simulink model "BAM"  (R2025b)
settings: Solver=FixedStepAuto  StartTime=0.0  StopTime=SimPar.model_params.stop_time  RelTol=1e-3
libraries: simulink x1
settings Model: Creator=macheson  LastModifiedBy=wyatt

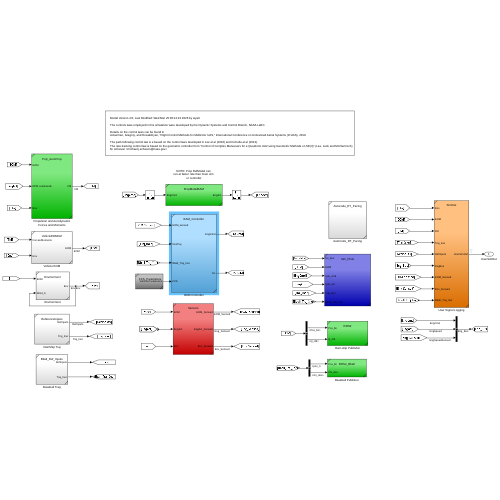
[thumbnail: Simulink's stored preview of the top-level diagram]
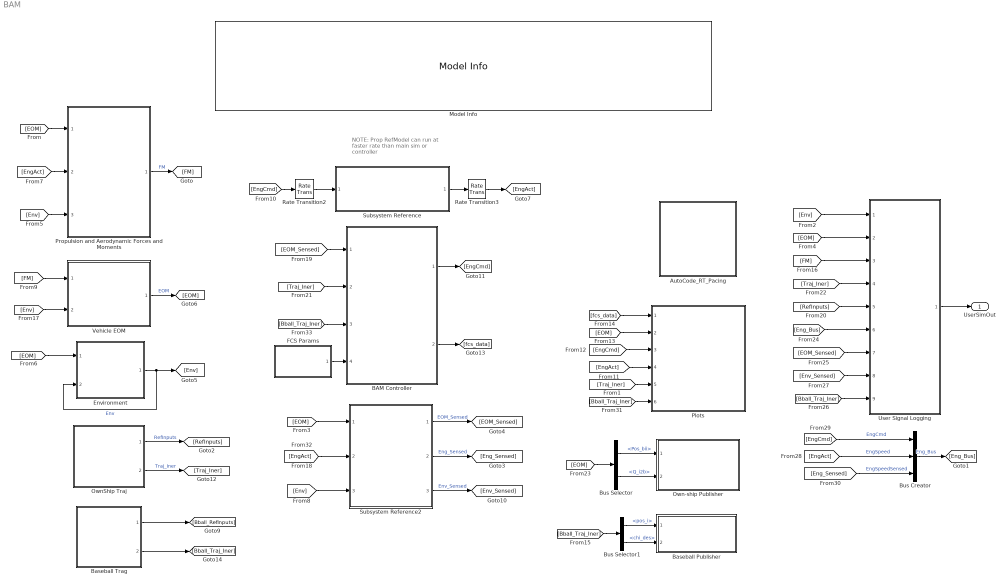
== system BAM ==
  note: NOTE: Prop RefModel can
      | run at faster rate than main sim
      | or controller
  AutoCode_RT_Pacing : Subsystem  ReferencedSubsystem=Autocode_RT_Pacing
  BAM Controller : Subsystem  ReferencedSubsystem=BAM_Controller
  Baseball Publisher : Subsystem  ReferencedSubsystem=ROS2_Bball
  Baseball Trag : Subsystem  ReferencedSubsystem=Bball_Ref_Inputs
  Bus Creator : BusCreator  Inputs=3  OutDataTypeStr=Bus: BUS_PROP_CMD
  Bus Selector : BusSelector  OutputSignals=InertialData.Pos_bii,InertialData.Q_i2b
  Bus Selector1 : BusSelector  OutputSignals=pos_i,chi_des
  Environment : Subsystem  ReferencedSubsystem=Environment
  FCS Params : Subsystem  ReferencedSubsystem=FCS_Parameters
  Model Info : simulink/Model-Wide Utilities/Model Info  Frame=on  DisplayStringWithTags=|  HorizontalTextAlignment=Left  LeftAlignmentValue=0.02
      | Model Version %<ModelVersion>; Last Modified: %<LastModificationDate> by %<LastModifiedBy>
      | 
      | The controls laws employed in this simulation were developed by the Dynamic Systems and Control Branch, NASA LaRC.
      | 
      | Details on the control laws can be found in
      | Ackerman, Gregory, and Hovakimyan, "Flight Control Methods for Multirotor UAS," International Conference on Unmanned Aerial Systems (ICUAS), 2019.
      | 
      | The path-following control law is a based on the control laws developed in Lee et al (2010) and Cichella et al (2013). 
      | The rate-tracking control law is based on the geometric controller from "Control of Complex Maneuvers for a Quadrotor UAV using Geometric Methods on SE(3)" (Lee, Leok and McClamroch)
      | M. Acheson <michael.j.acheson@nasa.gov>
  Own-ship Publisher : Subsystem  ReferencedSubsystem=ROS2
  OwnShip Traj : Subsystem  ReferencedSubsystem=ReferenceInputs
  Plots : Subsystem  ReferencedSubsystem=Sim_Plots
  Propulsion and Aerodynamic Forces and Moments : Subsystem  ReferencedSubsystem=Poly_AeroProp
  Rate Transition2 : RateTransition  OutPortSampleTime=SimIn.model_params.sim_rate
  Rate Transition3 : RateTransition  OutPortSampleTime=SimIn.model_params.sim_rate
  Subsystem Reference : Subsystem  ReferencedSubsystem=PropModelBAM
  Subsystem Reference2 : Subsystem  ReferencedSubsystem=Sensors
  User Signal Logging : Subsystem  ReferencedSubsystem=SimOut
  Vehicle EOM : Subsystem  ReferencedSubsystem=VehicleEOMRef
  UserSimOut : Outport
  wires:
  Vehicle EOM/1 -> [EOM]  "EOM"
  [FM] -> Vehicle EOM/1
  [Env] -> Vehicle EOM/2
  [EOM] -> Propulsion and Aerodynamic Forces and Moments/1
  OwnShip Traj/1 -> [RefInputs]  "RefInputs"
  Propulsion and Aerodynamic Forces and Moments/1 -> [FM]  "FM"
  [EOM] -> Subsystem Reference2/1
  Environment/1 -> Environment/2, [Env]  "Env"
  [EOM] -> Environment/1
  Subsystem Reference/1 -> Rate Transition3/1
  [EngCmd] -> Rate Transition2/1
  [EngAct] -> Plots/4
  [EngCmd] -> Plots/3
  [EOM] -> Plots/2
  [fcs_data] -> Plots/1
  [EngAct] -> Propulsion and Aerodynamic Forces and Moments/2
  Rate Transition2/1 -> Subsystem Reference/1
  Rate Transition3/1 -> [EngAct]
  Subsystem Reference2/2 -> [Eng_Sensed]  "Eng_Sensed"
  Subsystem Reference2/3 -> [Env_Sensed]  "Env_Sensed"
  [Env] -> Subsystem Reference2/3
  [EngAct] -> Subsystem Reference2/2
  Subsystem Reference2/1 -> [EOM_Sensed]  "EOM_Sensed"
  FCS Params/1 -> BAM Controller/4
  [EOM_Sensed] -> BAM Controller/1
  [Traj_Iner] -> BAM Controller/2
  BAM Controller/1 -> [EngCmd]
  OwnShip Traj/2 -> [Traj_Iner]  "Traj_Iner"
  BAM Controller/2 -> [fcs_data]
  [Env] -> User Signal Logging/1
  [EOM] -> User Signal Logging/2
  [Env_Sensed] -> User Signal Logging/8
  [EOM_Sensed] -> User Signal Logging/7
  [Eng_Bus] -> User Signal Logging/6
  [Traj_Iner] -> User Signal Logging/4
  [RefInputs] -> User Signal Logging/5
  [FM] -> User Signal Logging/3
  Bus Creator/1 -> [Eng_Bus]  "Eng_Bus"
  [Eng_Sensed] -> Bus Creator/3  "EngSpeedSensed"
  [EngAct] -> Bus Creator/2  "EngSpeed"
  [EngCmd] -> Bus Creator/1  "EngCmd"
  [EOM] -> Bus Selector/1
  Bus Selector/1 -> Own-ship Publisher/1  "<Pos_bii>"
  Bus Selector/2 -> Own-ship Publisher/2  "<Q_i2b>"
  User Signal Logging/1 -> UserSimOut/1
  [Traj_Iner] -> Plots/5
  Baseball Trag/1 -> [Bball_RefInputs]
  Baseball Trag/2 -> [Bball_Traj_Iner]
  [Bball_Traj_Iner] -> Plots/6
  [Bball_Traj_Iner] -> User Signal Logging/9
  [Bball_Traj_Iner] -> Bus Selector1/1
  Bus Selector1/1 -> Baseball Publisher/1  "<pos_i>"
  Bus Selector1/2 -> Baseball Publisher/2  "<chi_des>"
  [Env] -> Propulsion and Aerodynamic Forces and Moments/3
  [Bball_Traj_Iner] -> BAM Controller/3
